simulink library "Ampere_Library"  (R2022b)
settings: Solver=FixedStepDiscrete  StartTime=0  StopTime=10.0  RelTol=1e-3  EnableMultiTasking=on
undefined symbols (not defined in the file or in its folder): A_INST_double, Dem_EventStatusType, ECU_AMBIENT_TEMPERATURE, SET_ECU_AMBIENT_TEMPERATURE, SlDemoSign, Std_ReturnType
libraries: simulink x13
(part 1 of 10)
settings Model: ModifiedByFormat=Florian LEVY  Creator=Florian LEVY  LastModifiedBy=Florian LEVY
settings SolverCC: AlgebraicLoopSolver=TrustRegion
settings DataIOCC: LimitDataPoints=on  SaveFormat=Array  ReturnWorkspaceOutputs=off
settings OptimizationCC: DefaultParameterBehavior=Inlined  EfficientFloat2IntCast=on  LifeSpan=inf
settings DebuggingCC: SignalInfNanChecking=error  SignalRangeChecking=error  ReadBeforeWriteMsg=EnableAllAsError  WriteAfterWriteMsg=EnableAllAsError  WriteAfterReadMsg=EnableAllAsError  AlgebraicLoopMsg=error  ArtificialAlgebraicLoopMsg=error  SaveWithDisabledLinksMsg=error  SaveWithParameterizedLinksMsg=error  BlockPriorityViolationMsg=error  MinStepSizeMsg=error  TimeAdjustmentMsg=warning  SolverPrmCheckMsg=error  TasksWithSamePriorityMsg=error  SigSpecEnsureSampleTimeMsg=error  CheckMatrixSingularityMsg=error  IntegerOverflowMsg=error  ParameterUnderflowMsg=error  ParameterPrecisionLossMsg=error  ParameterTunabilityLossMsg=error  UnderSpecifiedDataTypeMsg=error  VectorMatrixConversionMsg=error  UnconnectedInputMsg=error  UnconnectedOutputMsg=error  UnconnectedLineMsg=error  UniqueDataStoreMsg=error  BusObjectLabelMismatch=error  RootOutportRequireBusObject=error  AssertControl=DisableAll  ModelReferenceIOMsg=error  UnknownTsInhSupMsg=error  ModelReferenceDataLoggingMessage=error  StateNameClashWarn=warning  StrictBusMsg=ErrorOnBusTreatedAsVector  NonBusSignalsTreatedAsBus=error  SFUnusedDataAndEventsDiag=error  SFInvalidInputDataAccessInChartInitDiag=error  SFTransitionOutsideNaturalParentDiag=error  SFUnreachableExecutionPathDiag=error  SFUndirectedBroadcastEventsDiag=error  SFTransitionActionBeforeConditionDiag=error  SFExecutionAtInitializationDiag=none  SFMachineParentedDataDiag=warning  ArithmeticOperatorsInVariantConditions=warning
settings HardwareCC: ProdBitPerPointer=32  ProdBitPerSizeT=32  ProdBitPerPtrDiffT=32  ProdLargestAtomicFloat=None  ProdIntDivRoundTo=Undefined  ProdEndianess=Unspecified  ProdWordSize=32  ProdHWDeviceType=32-bit Generic
settings ModelReferenceCC: EnableRefExpFcnMdlSchedulingChecks=on  PropagateSignalLabelsOutOfModel=off
settings SFSimCC: SimUseLocalCustomCode=off  CustomCodeUndefinedFunction=UseInterfaceOnly
settings RTWCC: RTWUseLocalCustomCode=off  DLArmComputeVersion=19.05
settings CodeAppCC: StateflowObjectComments=on
settings GRTTargetCC: TargetLangStandard=C89/C90 (ANSI)
settings ConfigComp: CovMetricSettings=dw  CovSaveCumulativeToWorkspaceVar=on  CovSaveSingleToWorkspaceVar=on  CovExternalEMLEnable=off

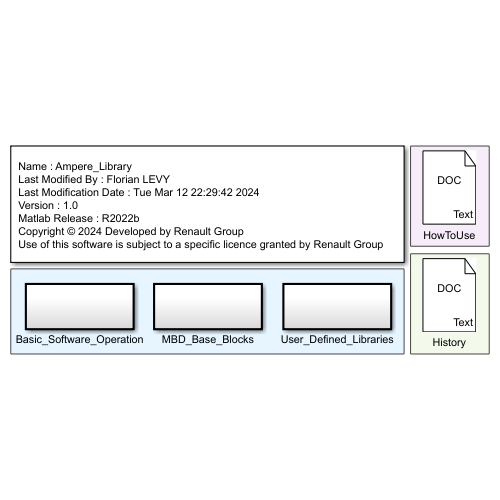
[thumbnail: Simulink's stored preview of the top-level diagram]
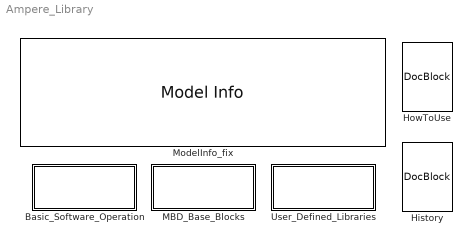
== system Ampere_Library ==
  Basic_Software_Operation : Subsystem  TreatAsAtomicUnit=on
  History : simulink/Model-Wide Utilities/DocBlock  DocumentType=Text
      content=|
      | Ampere Library V1.0 [12-Mar-2024]
      | - Creation of the library
      | - Creation of the block A_EnumConstant in User_Defined_Libraries/Sources to enhance model readability when using enumerated constants
  HowToUse : simulink/Model-Wide Utilities/DocBlock  DocumentType=Text
      content=|
      | This library contains 3 main sections:
      | - Basic_Software_Operation:
      |   Custom blocks to call operations such as DEM (cf rule CD059).
      |   For details about each block, refer to the documentations in their matching masks (double-click on the block).
      |
      | - MBD_Base_Blocks:
      |   Native Simulink blocks allowed by the LB001 rule.
      |   Eash subsections (Discrete, Sinks, etc..) contains copies from the native simulink library.
      |   All those blocks are directly configured as expected to be in compliance with the rules (e.g rule TY005, TY011, LK005, etc...).
      |
      | - User_Defined_Libraries:
      |   Custom blocks, most of them legacy, performing different operations such as delays, timers, detect changes, etc...
      |   For details about each block, refer to the documentations in their matching masks (double-click on the block).
      |
      | For more details, refer to the associated AMBD_Library_ReleaseNotes.pdf document.
      |
      | Notes:
      |  1) All custom blocks have:
      |    - a yellow backgrouncolor (authorized by LK013 rule)
      |    - a mask and the tag [LIB] (cf LB002 rule)
      |
      |  2) The library blocks are matching quality and process expectations, such as:
      |    - Readibility of all views
      |    - Data Flow easily identifiable (ex: Appropriate use of colors, cf rule LK013).
      |    - Mask callbacks optimized and commented
      |    - Compliance with Modelling rules and Metrics applicable at subsystem levels (ex: MT003, MT004, MT005)
      |
      |    => refer to:
      |       ASWP Unit Model Construction process
      |       Ampere Modelling Rules
  MBD_Base_Blocks : Subsystem  TreatAsAtomicUnit=on
  ModelInfo_fix : simulink/Model-Wide Utilities/Model Info  Frame=on  DisplayStringWithTags=|  HorizontalTextAlignment=Left  LeftAlignmentValue=0.02
      | Name : %<ModelName>
      | Last Modified By : Florian LEVY
      | Last Modification Date : %<LastModificationDate>
      | Version : 1.0
      | Matlab Release : R2022b
      | Copyright © 2024 Developed by Renault Group
      | Use of this software is subject to a specific licence granted by Renault Group
  User_Defined_Libraries : Subsystem  TreatAsAtomicUnit=on

== system Ampere_Library/Basic_Software_Operation ==
  note: Basic Software Operations
  Diagnostic_Event_Manager : Subsystem  TreatAsAtomicUnit=on
  HW_IO : Subsystem  TreatAsAtomicUnit=on

== system Ampere_Library/MBD_Base_Blocks ==
  note: Basic Simulink and Stateflow Blocks
  Simulink : Subsystem  TreatAsAtomicUnit=on
  Stateflow : Subsystem  TreatAsAtomicUnit=on

== system Ampere_Library/User_Defined_Libraries ==
  note: Functional Library Blocks
  Discontinuities : Subsystem  TreatAsAtomicUnit=on
  Discrete : Subsystem  TreatAsAtomicUnit=on
  FlipFlop : Subsystem  TreatAsAtomicUnit=on
  Logic_and_Bit_Operations : Subsystem  TreatAsAtomicUnit=on
  Lookup_Tables : Subsystem  TreatAsAtomicUnit=on
  Math_Operations : Subsystem  TreatAsAtomicUnit=on
  Miscellaneous : Subsystem  TreatAsAtomicUnit=on
  Signal_Routing : Subsystem  TreatAsAtomicUnit=on
  Sources : Subsystem  TreatAsAtomicUnit=on
  Timers_and_Counters : Subsystem  TreatAsAtomicUnit=on

== system Ampere_Library/Basic_Software_Operation/Diagnostic_Event_Manager ==
  note: Diagnostic Event Management Blocks
  A_ReportDiagnosticTestResult : Subsystem  Tag=[LIB]  mask(A_ReportDiagnosticTestResult){MonitoredComponent=DEVICE2, FaultType=SC_TO_GND3, DebounceAlgorithm=AUTOSAR}
      mask prompts: MonitoredComponent "Monitored Component"; FaultType "Fault Type"; DebounceAlgorithm "Debounce Algorithm"
      mask help:
      | This block reports the result of a diagnostic test to the BSW Diagnostic Event Manager,which is in charge of handling DTC-related operations based on this test result.The input is a boolean, with value 'true' indicating that a fault occurred.
      |
      | If "Debounce Algorithm" parameter is set to "AUTOSAR", test result will be further debounced by Basic SW, before being qualified as failed or not, according the UDS (ISO14229) definition.
      |
      | If "Debounce Algorithm" parameter is set to "specific", a test result will be considered as failed, according to the UDS (ISO 14229) definition as soon as the input is set to 'true'.
      |
      | A model that contains this block can not be simulated directly. It must be run through a harness model that contains a stub of the function that is called.
      |
      | Block parameters values are defined during the architecture stage.
      |
      | Monitored Component: Indicates the part or function to which the fault is attached.
      | Fault Type: Indicates the kind of fault
      | Debounce Algorithm: Indicates if debounce shall be performed by Applicative SW or Basic SW.
      mask init:
      | %% Initialization
      | try
      |     % Test if the enum Dem_EventStatusType already exists (loaded from a sldd or
      |     % the base workspace)
      |     Dem_EventStatusType.DEM_EVENT_STATUS_PASSED;
      | catch
      |     % Define the enum Dem_EventStatusType if not existing.
      |     Simulink.defineIntEnumType( 'Dem_EventStatusType', ...
      |         {'DEM_EVENT_STATUS_PASSED','DEM_EVENT_STATUS_FAILED','DEM_EVENT_STATUS_PREPASSED','DEM_EVENT_STATUS_PREFAILED'}, ...
      |         [0 1 2 3], ...
      |         'DefaultValue', 'DEM_EVENT_STATUS_PASSED', ...
      |         'StorageType', 'uint8', ...
      |         'HeaderFile', 'Rte_Type.h', ...
      |         'AddClassNameToEnumNames', false);
      | end
      | 
      | %% Set Block Parameters
      | MonitoredComponent_str = get_param(gcb,'MonitoredComponent');
      | FaultType_str = get_param(gcb,'FaultType');
      | 
      | % Update Constant blocks
      | if DebounceAlgorithm==1
      |      % Case Specific
      |     set_param([gcb '/DEM_EVENT_STATUS_F'],'Value','Dem_EventStatusType.DEM_EVENT_STATUS_FAILED');
      |     set_param([gcb '/DEM_EVENT_STATUS_P'],'Value','Dem_EventStatusType.DEM_EVENT_STATUS_PASSED');
      | else % DebounceAlgorithm==2
      |     % Case AUTOSAR
      |     set_param([gcb '/DEM_EVENT_STATUS_F'],'Value','Dem_EventStatusType.DEM_EVENT_STATUS_PREFAILED');
      |     set_param([gcb '/DEM_EVENT_STATUS_P'],'Value','Dem_EventStatusType.DEM_EVENT_STATUS_PREPASSED');
      | end
      | 
      | % Update FunctionCaller block
      | set_param([gcb '/DemSetEventStatusCall'],'FunctionPrototype',...
      |     sprintf('ERR=%s_%s_setEventStatus(EventStatus)',MonitoredComponent_str,FaultType_str));
      settings: AttributesFormatString=%<MaskType>
      mask Help: eval('specFile = ''A_ReportDiagnosticTestResult.pdf'';if isempty(which(specFile));warndlg(strcat(''Specification file : '',specFile, '' is not found. Please do addpath of "SPEC" folder which is present in the location where the Library resides''), ''Specification file not found'');else;open(specFile);end;clear specFile;');
      mask TypeOptions DebounceAlgorithm: Specific | AUTOSAR
      mask Display:
      | %% Display info on the icon
      | fprintf('Component: %s\nFault type: %s',MonitoredComponent_str,FaultType_str)

== system Ampere_Library/Basic_Software_Operation/HW_IO ==
  note: Those 3 blocks create data named
      | "A_INST_xxx" sent in the Base Workspace,
      | and used to defined the prototype of the
      | internal functioncallers.
  note: Hardware and I/O Operations
  A_HWDiag : Subsystem  Tag=[LIB]  mask(A_HWDiag){Signal_name=AMBIENT_TEMPERATURE, Signal_type=double}
      mask prompts: Signal_name "Symbolic HW Name"; Signal_type "Signal type"
      mask help:
      | This subsystem represents a call to the Basic Software, in order to retrieve the diagnostic status of an output of the ECU.
      |
      | A model that contains this block can not be simulated directly. It must be run through a harness model that contains a stub of the function that is called.
      |
      | Mask properties are defined during the architecture stage:
      |
      | 'Symbolic HW Name' represents the symbolic name of the HW Pin of the ECU whose diagnostic status is retrieved.
      |
      | 'Signal Type" represents the type of the output of the I/O HW Abstraction Layer module.
      |
      | WARNING: this block's callback creates a data "A_INST_xxx" in the base workspace.
      mask init:
      | %% Initialize Std_ReturnType
      | % Purpose: To support enumeration dependency if it is not available
      | try
      |     % Test if the enum Std_ReturnType already exists (loaded from a sldd or
      |     % the base workspace)
      |     Std_ReturnType.RTE_E_OK;
      | catch
      |     % Define the enum Std_ReturnType if not existing.
      |     Simulink.defineIntEnumType('Std_ReturnType', ...
      |         {'RTE_E_OK', 'RTE_E_INVALID'}, ...
      |         [0;1], ...
      |         'Description', 'Standard error codes according to SWS_Std_00005. This description has been user-defined, not SIMULINK-generated', ...
      |         'DefaultValue', 'RTE_E_OK', ...
      |         'HeaderFile', 'Rte_Type.h', ...
      |         'DataScope', 'Auto', ...
      |         'StorageType', 'uint8');
      | end
      | 
      | %% Get signal name
      | Signal_name_str = get_param(gcb,'Signal_name');
      | % Name to put on the outport
      | Outport_nm = ['ECU_' Signal_name_str '_dg'];
      | 
      | %% Callback routine
      | Sig_type_str = get_param(gcb,'Signal_type');
      | Inst_Data = Simulink.Parameter;
      | 
      | % Create the name and default value of the Parameter that will be created in the base
      | % workspace : "A_INST_" + appropriate datatype
      | if ~isempty(regexpi(Sig_type_str,'^Enum:','once'))
      |     % Case Enums
      |     Enum_split_cell = regexpi(Sig_type_str,'Enum:','split');
      |     Enum_split_cell = Enum_split_cell(~cellfun('isempty',Enum_split_cell));
      |     Enum_DT = Enum_split_cell{end};
      |     Enum_DT = regexprep(Enum_DT,' ','');
      |     Enum_object = enumeration(Enum_DT);
      |     if ~isempty(Enum_object)
      |         Inst_value = Enum_object(1);
      |     else
      |         error('Define a valid enumeration class for Signal type parameter.')
      |     end
      |     Instant_var_str = ['A_INST_' Enum_DT];
      | 
      | elseif ~isempty(regexpi(Sig_type_str,'^fixdt(','once'))
      |     % Case fixdt
      |     Inst_value = 0;
      |     Instant_var_str = ['A_INST_' 'fixdt'];
      | 
      | else
      |     % Other cases 
      |     Inst_value = 0;
      |     Instant_var_str = ['A_INST_' Sig_type_str];
      |     
      | end
      | Inst_Data.DataType = Sig_type_str;
      | Inst_Data.Value = Inst_value;
      | 
      | % send the parameter object in the base workspace
      | assignin('base', Instant_var_str, Inst_Data);
      | 
      | %% Update internal blocks
      | % Update the functioncaller block prototype
      | set_param([gcb '/PhysicalSampling'],...
      |     'FunctionPrototype' , ['[ECU_' Signal_name_str '_dg,RTE_Error] = GET_DIAG_' Signal_name_str '()'],...
      |     'OutputArgumentSpecifications' , [ Instant_var_str '(1),Std_ReturnType(1)']);
      | 
      | % Update the outport 1 name and datatype
      | set_param(char(find_system(gcb,'FollowLinks','on','LookUnderMasks','all','Blocktype','Outport','Port','1')),...
      |     'Name' , Outport_nm,...
      |     'OutDataTypeStr' , get_param(gcb,'Signal_type'));
      settings: AttributesFormatString=|
      | %<MaskType>
      | Signal type = %<Signal_type>
      mask Help: eval('specFile = ''A_HWDiag.pdf'';if isempty(which(specFile));warndlg(strcat(''Specification file : '',specFile, '' is not found. Please do addpath of "SPEC" folder which is present in the location where the Library resides''), ''Specification file not found'');else;open(specFile);end;clear specFile;');
      mask Display:
      | %% Display info on the icon
      | color('blue');
      | text(.5,.5,'ECU_"SymbolName"_dg','HorizontalAlignment','center');
  A_HWInput : Subsystem  Tag=[LIB]  mask(A_HWInput){Signal_name=AMBIENT_TEMPERATURE, Signal_type=double}
      mask prompts: Signal_name "Symbolic HW Name"; Signal_type "Signal type"
      mask help:
      | This subsystem represents a call to the Basic Software, in order to get the value of the data from the ECU input stage.
      |
      | A model that contains this block can not be simulated directly. It must be run through a harness model that contains a stub of the function that is called.
      |
      | Mask properties are defined during the architecture stage:
      |
      | 'Symbolic HW Name' represents the symbolic name of the HW Pin of the ECU that is read.
      |
      | 'Signal Type" represents the type of the output of the I/O HW Abstraction Layer module.
      |
      | WARNING: this block's callback creates a data "A_INST_xxx" in the base workspace.
      mask init:
      | %% Initialize Std_ReturnType
      | % Purpose: To support enumeration dependency if it is not available
      | try
      |     % Test if the enum Std_ReturnType already exists (loaded from a sldd or
      |     % the base workspace)
      |     Std_ReturnType.RTE_E_OK;
      | catch
      |     Simulink.defineIntEnumType('Std_ReturnType', ...
      |     	{'RTE_E_OK', 'RTE_E_INVALID'}, ...
      |     	[0;1], ...
      |     	'Description', 'Standard error codes according to SWS_Std_00005. This description has been user-defined, not SIMULINK-generated', ...
      |     	'DefaultValue', 'RTE_E_OK', ...
      |     	'HeaderFile', 'Rte_Type.h', ...
      |     	'DataScope', 'Auto', ...
      |     	'StorageType', 'uint8');
      | end
      | 
      | %% Get signal name
      | Signal_name_str = get_param(gcb,'Signal_name');
      | % Name to put on the outport
      | Outport_nm = ['ECU_' Signal_name_str];
      | 
      | %% Callback routine
      | Sig_type_str = get_param(gcb,'Signal_type');
      | Inst_Data = Simulink.Parameter;
      | 
      | % Create the name and default value of the Parameter that will be created in the base
      | % workspace : "A_INST_" + appropriate datatype
      | if ~isempty(regexpi(Sig_type_str,'^Enum:','once'))
      |     % Case Enums
      |     Enum_split_cell = regexpi(Sig_type_str,'Enum:','split');
      |     Enum_split_cell = Enum_split_cell(~cellfun('isempty',Enum_split_cell));
      |     Enum_DT = Enum_split_cell{end};
      |     Enum_DT = regexprep(Enum_DT,' ','');
      |     Enum_object = enumeration(Enum_DT);
      |     if ~isempty(Enum_object)
      |         Inst_value = Enum_object(1);
      |     else
      |         error('Define a valid enumeration class for Signal type parameter.')
      |     end
      | 
      |     Instant_var_str = ['A_INST_' Enum_DT];
      | 
      | elseif ~isempty(regexpi(Sig_type_str,'^fixdt(','once'))
      |     % Case fixd
      |     Inst_value = 0;
      |     Instant_var_str = ['A_INST_' 'fixdt'];
      | 
      | else
      |     % Other cases
      |     Inst_value = 0;
      |     Instant_var_str = ['A_INST_' Sig_type_str];
      | end
      | Inst_Data.DataType = Sig_type_str;
      | Inst_Data.Value = Inst_value;
      | 
      | % send the parameter object in the base workspace
      | assignin('base', Instant_var_str, Inst_Data);
      | 
      | %% Update internal blocks
      | % Update the functioncaller block prototype
      | set_param([gcb '/PhysicalSampling'],...
      |     'FunctionPrototype' , ['[ECU_' Signal_name_str ',RTE_Error] = GET_ECU_' Signal_name_str '()'],...
      |     'OutputArgumentSpecifications' , [ Instant_var_str '(1),Std_ReturnType(1)']);
      | 
      | % Update the outport 1 name and datatype
      | set_param(char(find_system(gcb,'FollowLinks','on','LookUnderMasks','all','Blocktype','Outport','Port','1')),...
      |     'Name' , Outport_nm,...
      |     'OutDataTypeStr' , get_param(gcb,'Signal_type'));
      settings: AttributesFormatString=|
      | %<MaskType>
      | Signal type = %<Signal_type>
      mask Help: eval('specFile = ''A_HWInput.pdf'';if isempty(which(specFile));warndlg(strcat(''Specification file : '',specFile, '' is not found. Please do addpath of "SPEC" folder which is present in the location where the Library resides''), ''Specification file not found'');else;open(specFile);end;clear specFile;');
      mask Display:
      | %% Display info on the icon
      | color('blue');
      | text(.5,.5,'ECU_"SymbolName"','HorizontalAlignment','center');
  A_HWOutput : Subsystem  Tag=[LIB]  mask(A_HWOutput){Signal_name=AMBIENT_TEMPERATURE, Signal_type=double}
      mask prompts: Signal_name "Symbolic HW Name"; Signal_type "Signal type"
      mask help:
      | This subsystem represents a call to the Basic Software, so as to set the value of an output of the ECU.
      |
      | A model that contains this block can not be simulated directly. It must be run through a harness model that contains a stub of the function that is called.
      |
      | Mask properties are defined during the architecture stage.
      |
      | 'Symbolic HW Name' represents the symbolic name of the HW Pin of the ECU that is set.
      |
      | 'Signal Type" represents the type of the output of the I/O HW Abstraction Layer module.
      |
      | WARNING: this block's callback creates a data "A_INST_xxx" in the base workspace.
      mask init:
      | %% Get signal name
      | Signal_name_str = get_param(gcb,'Signal_name');
      | % Name to put on the Inport
      | Inport_nm = ['ECU_' Signal_name_str];
      | 
      | %% Callback routine
      | Sig_type_str = get_param(gcb,'Signal_type');
      | Inst_Data = Simulink.Parameter;
      | 
      | % Create the name and default value of the Parameter that will be created in the base
      | % workspace : "A_INST_" + appropriate datatype
      | if ~isempty(regexpi(Sig_type_str,'^Enum:','once'))
      |     % Case Enums
      |     Enum_split_cell = regexpi(Sig_type_str,'Enum:','split');
      |     Enum_split_cell = Enum_split_cell(~cellfun('isempty',Enum_split_cell));
      |     Enum_DT = Enum_split_cell{end};
      |     Enum_DT = regexprep(Enum_DT,' ','');
      |     Enum_object = enumeration(Enum_DT);
      |     if ~isempty(Enum_object)
      |         Inst_value = Enum_object(1);
      |     else
      |         error('Define a valid enumeration class for Signal type parameter.')
      |     end
      |     Instant_var_str = ['A_INST_' Enum_DT];
      | 
      | elseif ~isempty(regexpi(Sig_type_str,'^fixdt(','once'))
      |     % Case fixdt
      |     Inst_value = 0;
      |     Instant_var_str = ['A_INST_' 'fixdt'];
      | else
      |     % Other cases
      |     Inst_value = 0;
      |     Instant_var_str = ['A_INST_' Sig_type_str];
      | end
      | Inst_Data.DataType = Sig_type_str;
      | Inst_Data.Value = Inst_value;
      | 
      | % send the parameter object in the base workspace
      | assignin('base', Instant_var_str, Inst_Data);
      | 
      | %% Update internal blocks
      | % Update the functioncaller block prototype
      | set_param([gcb '/PhysicalSampling'],...
      |     'FunctionPrototype',['SET_ECU_' Signal_name_str '(ECU_' Signal_name_str ')'],...
      |     'InputArgumentSpecifications',[ Instant_var_str '(1)']);
      | 
      | % Update the inport 1 name
      | set_param(char(find_system(gcb,'FollowLinks','on','LookUnderMasks','all','Blocktype','Inport','Port','1')),...
      |     'Name',Inport_nm);
      settings: AttributesFormatString=|
      | %<MaskType>
      | Signal type = %<Signal_type>
      mask Help: eval('specFile = ''A_HWOutput.pdf'';if isempty(which(specFile));warndlg(strcat(''Specification file : '',specFile, '' is not found. Please do addpath of "SPEC" folder which is present in the location where the Library resides''), ''Specification file not found'');else;open(specFile);end;clear specFile;');
      mask Display:
      | %% Display info on the icon
      | color('blue');
      | text(.5,.85,'ECU_"SymbolName"','HorizontalAlignment','center');

== system Ampere_Library/MBD_Base_Blocks/Simulink ==
  note: Basic Simulink Blocks
  CommonlyUsedBlocks : Subsystem  TreatAsAtomicUnit=on
  Discontinuities : Subsystem  TreatAsAtomicUnit=on
  Discrete : Subsystem  TreatAsAtomicUnit=on
  Logic_and_Bit_Operations : Subsystem  TreatAsAtomicUnit=on
  Lookup_Tables : Subsystem  TreatAsAtomicUnit=on
  Math_Operations : Subsystem  TreatAsAtomicUnit=on
  Model_Wide_Utilities : Subsystem  TreatAsAtomicUnit=on
  Ports_and_Subsystems : Subsystem
  Signal_Attributes : Subsystem  TreatAsAtomicUnit=on
  Signal_Routing : Subsystem  TreatAsAtomicUnit=on
  Sinks : Subsystem  TreatAsAtomicUnit=on
  Sources : Subsystem  TreatAsAtomicUnit=on
  User_Defined_Functions : Subsystem  TreatAsAtomicUnit=on

== system Ampere_Library/MBD_Base_Blocks/Stateflow ==
  note: Stateflow
  Chart : Stateflow chart  TreatAsAtomicUnit=on
      settings: CopyFcn=set_param(gcbh,'LinkStatus','none'); set_param(gcbh,'Mask','off'); set_param(gcbh,'MaskType',''); set_param(gcbh,'MaskDescription',''); set_param(gcbh,'OpenFcn',''); set_param(gcbh,'CopyFcn','');  OpenFcn=open_system(gcbh,'force');
